simulink model "pr662_pll2_noise"  (R2018b)
settings: Solver=VariableStepDiscrete  StartTime=0.0  StopTime=(n-1)*T  RelTol=1e-3  EnableMultiTasking=on
PreLoadFcn:
  | pr662_configure_pll2;
StartFcn:
  | close all;
values from neighbouring files (symbols this model uses):
  awgn = 0.05    [pr662_configure_pll2.m]
  ferr = 4500    [pr662_configure_pll2.m]
  fq = 1e6    (= 1000000)    [pr662_configure_pll2.m]
  fs = 10e6    (= 10000000)    [pr662_configure_pll2.m]
  K1 = (4*d*eta)/(Ko*Kp*(1+(2*d*eta)+eta^2))    (= 0.0106371918588)    [pr662_configure_pll2.m]
  K2 = (4*eta^2)/(Ko*Kp*(1+(2*d*eta)+eta^2))    (= 2.83715570971e-05)    [pr662_configure_pll2.m]
  Ko = 1    [pr662_configure_pll2.m]
Description:
  | Software, Simulation Examples and Design Exercises Licence Agreement
  | 
  | This license agreement refers to the simulation examples, design exercises and files,
  | and associated software MATLAB and Simulink resources that accompany the book:
  | 
  |      Title: Software Defined Radio using MATLAB & Simulink and the RTL-SDR
  |      Published by Strathclyde Academic Media, 2015
  |      Authored by Robert W. Stewart, Kenneth W. Barlee, Dale S.W. Atkinson,
  |      and Louise H. Crockett
  | 
  | and made available as a download from, www.desktopSDR.com or variously acquired
  | by other means such as via USB storage, cloud storage, disk or any other electronic
  | or optical or magnetic storage mechanism. These files and associated software may
  | be used subject to the terms of agreement of the conditions below:
  | 
  |     Copyright © 2015 Robert W. Stewart, Kenneth W. Barlee, Dale S.W. Atkinson,
  |     and Louise H. Crockett
  |     All rights reserved.
  | 
  | Redistribution and use in source and binary forms, with or without modification, are
  | permitted provided that the following conditions are met:
  | 
  |    1.  Redistributions of source code must retain the above copyright notice, this list of
  |         conditions and the following disclaimer.
  | 
  |    2.  Redistributions in binary form must reproduce the above copyright notice, this
  |         list of conditions and the following disclaimer in the documentation and/or other
  |         materials provided with the distribution.
  | 
  |    3.  Neither the name of the copyright holder nor the names of its contributors may
  |         be used to endorse or promote products derived from this software without
  |         specific prior written permission.
  | 
  |    4.  In all cases, the software is, and all modifications and derivatives of the
  |         software shall be, licensed to you solely for use in conjunction with The
  |         MathWorks, Inc. products and service offerings.
  | 
  | THIS SOFTWARE IS PROVIDED BY THE COPYRIGHT HOLDERS AND CONTRIBUTORS
  | "AS IS" AND ANY EXPRESS OR IMPLIED WARRANTIES, INCLUDING, BUT NOT LIMITED
  | TO, THE IMPLIED WARRANTIES OF MERCHANTABILITY AND FITNESS FOR A
  | PARTICULAR PURPOSE ARE DISCLAIMED. IN NO EVENT SHALL THE COPYRIGHT
  | HOLDER OR CONTRIBUTORS BE LIABLE FOR ANY DIRECT, INDIRECT, INCIDENTAL,
  | SPECIAL, EXEMPLARY, OR CONSEQUENTIAL DAMAGES (INCLUDING, BUT NOT
  | LIMITED TO, PROCUREMENT OF SUBSTITUTE GOODS OR SERVICES; LOSS OF USE,
  | DATA, OR PROFITS; OR BUSINESS INTERRUPTION) HOWEVER CAUSED AND ON ANY
  | THEORY OF LIABILITY, WHETHER IN CONTRACT, STRICT LIABILITY, OR TORT
  | (INCLUDING NEGLIGENCE OR OTHERWISE) ARISING IN ANY WAY OUT OF THE USE
  | OF THIS SOFTWARE, EVEN IF ADVISED OF THE POSSIBILITY OF SUCH DAMAGE.
  | 
  | 
  | Audio Tracks used in Simulations Examples and Design Exercises
  | 
  | The music and vocal files used within the Examples files and software within the book
  | were variously written, arranged, performed, recorded and produced by Garrey Rice,
  | Adam Struth, Jamie Struth, Iain Thistlethwaite and also Marshall Craigmyle who
  | collectively, and individually where appropriate, assert and retain all of their copyright,
  | performance and artistic rights. Permission to use and reproduce this music is
  | granted for all purposes associated with MATLAB and Simulink software and the
  | simulation examples and design exercises files that accompany this book. Requests to
  | use the music for any other purpose should be directed to: info@desktopSDR.com.
  | For information on music track names, full credits, and links to the musicians please
  | refer to www.desktopSDR.com/more/audio.
settings Model: Creator=desktopSDR Team  LastModifiedBy=Григорий Фокин
settings DataIOCC: SaveFormat=Array  SaveOutput=off  SignalLogging=off  SaveTime=off
settings OptimizationCC: LifeSpan=inf
settings DebuggingCC: UnderspecifiedInitializationDetection=Classic  MergeDetectMultiDrivingBlocksExec=none  SolverPrmCheckMsg=warning  SFUnexpectedBacktrackingDiag=warning  SFNoUnconditionalDefaultTransitionDiag=warning  SFExecutionAtInitializationDiag=none
settings HardwareCC: ProdBitPerPointer=32  ProdBitPerSizeT=32  ProdBitPerPtrDiffT=32  ProdLargestAtomicFloat=None  ProdIntDivRoundTo=Undefined  ProdEndianess=Unspecified  ProdWordSize=32  ProdHWDeviceType=32-bit Generic
settings ModelReferenceCC: PropagateSignalLabelsOutOfModel=off
settings SFSimCC: SimUseLocalCustomCode=off
settings RTWCC: RTWUseLocalCustomCode=off
settings CodeAppCC: StateflowObjectComments=on
settings GRTTargetCC: TargetLangStandard=C89/C90 (ANSI)  GeneratePreprocessorConditionals=Disable all
settings ConfigComp: CovMetricSettings=dw  CovHtmlReporting=on  CovSaveCumulativeToWorkspaceVar=on  CovSaveSingleToWorkspaceVar=on  CovExternalEMLEnable=off  CovSFcnEnable=off

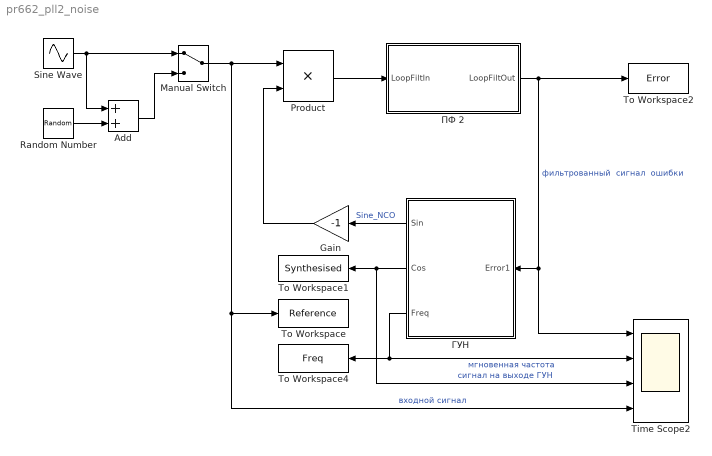
== system pr662_pll2_noise ==
  Add : Sum
  Gain : Gain  Gain=-1
  Manual Switch : ManualSwitch
  Product : Product
  Random Number : RandomNumber  Variance=awgn  SampleTime=1/fs
  Sine Wave : Sin  Frequency=2*pi*(fq+ferr)  Phase=pi/5  SampleTime=0
  Time Scope2 : Scope  NumInputPorts=4
  To Workspace : ToWorkspace  VariableName=Reference  SampleTime=-1
  To Workspace1 : ToWorkspace  VariableName=Synthesised  SampleTime=-1
  To Workspace2 : ToWorkspace  VariableName=Error  SampleTime=-1
  To Workspace4 : ToWorkspace  VariableName=Freq  SampleTime=-1
  ГУН : Subsystem
  ПФ 2 : Subsystem  mask(Loop Filter (Type 2)){K1=K1, K2=K2}
      mask prompts: K1 "K1 (proportional path)"; K2 "K2 (integral path)"
      mask help: This loop filter contains two paths: a proportional path with scaling coefficient K1, and an integral path with scaling coefficient K2.
  wires:
  Manual Switch/1 -> Time Scope2/4, To Workspace/1, Product/1  "входной сигнал"
  ПФ 2/1(LoopFiltOut) -> To Workspace2/1, Time Scope2/1, ГУН/1(Error1)  "фильтрованный  сигнал  ошибки"
  Sine Wave/1 -> Add/1, Manual Switch/1
  ГУН/2(Cos) -> To Workspace1/1, Time Scope2/3  "сигнал на выходе ГУН"
  Product/1 -> ПФ 2/1(LoopFiltIn)
  Add/1 -> Manual Switch/2
  Random Number/1 -> Add/2
  ГУН/3(Freq) -> Time Scope2/2, To Workspace4/1  "мгновенная частота"
  ГУН/1(Sin) -> Gain/1  "Sine_NCO"
  Gain/1 -> Product/2

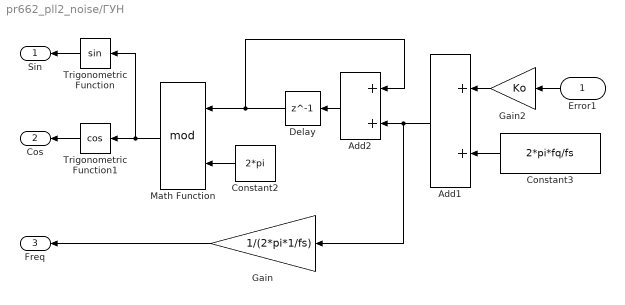
== system pr662_pll2_noise/ГУН ==
  Error1 : Inport
  Add1 : Sum  AccumDataTypeStr=single
  Add2 : Sum  AccumDataTypeStr=single
  Constant2 : Constant  Value=2*pi  OutDataTypeStr=double
  Constant3 : Constant  Value=2*pi*fq/fs  OutDataTypeStr=double
  Delay : Delay  DelayLength=1  InitialCondition=0.001
  Gain : Gain  Gain=1/(2*pi*1/fs)
  Gain2 : Gain  Gain=Ko  OutDataTypeStr=single
  Math Function : Math  Operator=mod  SaturateOnIntegerOverflow=on
  Trigonometric Function : Trigonometry
  Trigonometric Function1 : Trigonometry  Operator=cos
  Sin : Outport
  Cos : Outport  Port=2
  Freq : Outport  Port=3
  wires:
  Gain/1 -> Freq/1
  Add1/1 -> Gain/1, Add2/2
  Add2/1 -> Delay/1
  Constant2/1 -> Math Function/2
  Trigonometric Function/1 -> Sin/1
  Math Function/1 -> Trigonometric Function/1, Trigonometric Function1/1
  Trigonometric Function1/1 -> Cos/1
  Constant3/1 -> Add1/2
  Delay/1 -> Add2/1, Math Function/1
  Error1/1 -> Gain2/1
  Gain2/1 -> Add1/1

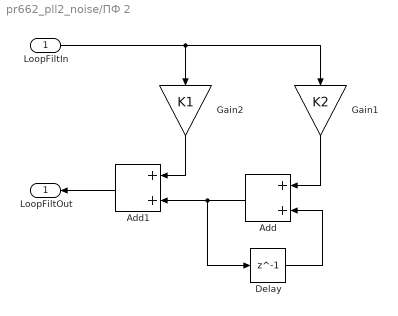
== system pr662_pll2_noise/ПФ 2 ==
  LoopFiltIn : Inport
  Add : Sum
  Add1 : Sum
  Delay : Delay  DelayLength=1
  Gain1 : Gain  Gain=K2
  Gain2 : Gain  Gain=K1
  LoopFiltOut : Outport
  wires:
  Add1/1 -> LoopFiltOut/1
  Delay/1 -> Add/2
  Add/1 -> Delay/1, Add1/2
  LoopFiltIn/1 -> Gain1/1, Gain2/1
  Gain2/1 -> Add1/1
  Gain1/1 -> Add/1
